simulink model "Kinematics"  (R2024a)
settings: Solver=VariableStepAuto  StartTime=0.0  StopTime=10.0  RelTol=1e-3
values from neighbouring files (symbols this model uses):
  Achsabstand = 0.15    [Model1Sensibilities.m]    (also in Model1numericalPSA.m; Model2Sensibilities.m; Modellvalidierung.m; MotorSens2.m)
  B_dis = 0.25    [Model1Sensibilities.m]    (also in Model1numericalPSA.m = 0.15; Model2Sensibilities.m; Modellvalidierung.m = 0.15; MotorSens2.m)
settings Model: Creator=jakob  LastModifiedBy=jakob

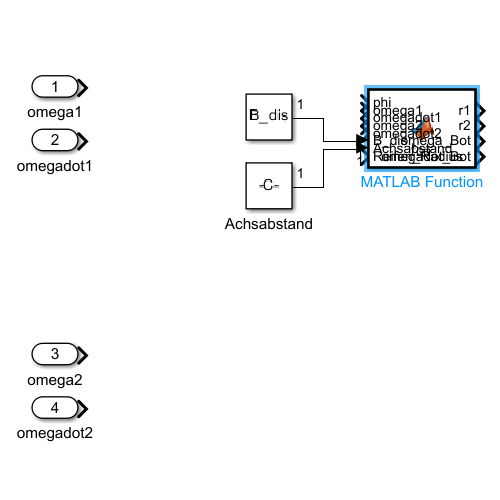
[thumbnail: Simulink's stored preview of the top-level diagram]
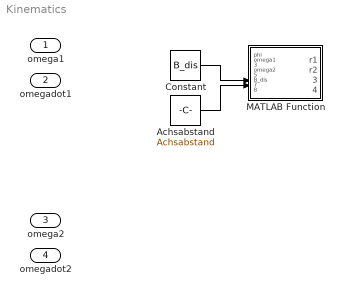
== system Kinematics ==
  omega1 : Inport
  omegadot1 : Inport  Port=2
  omega2 : Inport  Port=3
  omegadot2 : Inport  Port=4
  Achsabstand : Constant  Value=Achsabstand
  Constant : Constant  Value=B_dis
  MATLAB Function : MATLAB Function  TreatAsAtomicUnit=on
  wires:
  Constant/1 -> MATLAB Function/6(B_dis)
  Achsabstand/1 -> MATLAB Function/7(Achsabstand)

== matlab function Kinematics/MATLAB Function ==
  data: phi input; omega1 input; omegadot1 input; omega2 input; omegadot2 input; r1 output; B_dis input; Achsabstand input; r2 output; Reifen_Radius input; omega_Bot output; omegadot_Bot output
function [r1, r2, omega_Bot, omegadot_Bot]= fcn(phi, omega1, omegadot1, omega2, omegadot2, B_dis, Achsabstand , Reifen_Radius)

r1x = (1/3)*cos(phi)* B_dis - (1/2)*sin(phi)*Achsabstand;
r1y = (1/3)*sin(phi)* B_dis + (1/2)*cos(phi)*Achsabstand;
r2x = (1/3)*cos(phi)* B_dis + (1/2)*sin(phi)*Achsabstand;
r2y = (1/3)*sin(phi)* B_dis - (1/2)*cos(phi)*Achsabstand;

r1 = [r1x ; r1y ; 0];
r2 = [r2x ; r2y ; 0];
deltar = r1-r2;

phivec = [cos(phi); sin(phi)];
v1 = phivec * omega1 * Reifen_Radius;
v2 = phivec * omega2 * Reifen_Radius;
a1 = phivec * omegadot1 * Reifen_Radius;
a2 = phivec * omegadot2 * Reifen_Radius;

Rot_r = [0 -deltar(3) deltar(2) ; deltar(3) 0 -deltar(1); -deltar(2) deltar(1) 0];
omega_Bot = linsolve(Rot_r, v2-v1);
omegadot_Bot = linsolve(Rot_r, a2-a1 - cross(omega_Bot,cross(omega_Bot, r2-r1)));
